simulink model "ModelSimulationOfTheRunningDeviationSystem"  (Simulink 8.9)
settings: Solver=VariableStepAuto  StartTime=0.0  StopTime=10.0  RelTol=1e-3
settings Model: Creator=xiang  LastModifiedBy=xiang
settings DataIOCC: LimitDataPoints=off  SaveFormat=Dataset  SignalLoggingSaveFormat=Dataset
settings OptimizationCC: LifeSpan=auto
settings DebuggingCC: UnderspecifiedInitializationDetection=Simplified  MergeDetectMultiDrivingBlocksExec=error  FcnCallInpInsideContextMsg=error  StateNameClashWarn=none  SFUnexpectedBacktrackingDiag=error  SFNoUnconditionalDefaultTransitionDiag=error  SFExecutionAtInitializationDiag=warning
settings HardwareCC: ProdBitPerPointer=64  ProdBitPerSizeT=64  ProdBitPerPtrDiffT=64  ProdLargestAtomicFloat=Float  ProdIntDivRoundTo=Zero  ProdEndianess=LittleEndian  ProdWordSize=64  ProdHWDeviceType=Intel->x86-64 (Windows64)
settings ModelReferenceCC: PropagateSignalLabelsOutOfModel=on
settings GRTTargetCC: TargetLangStandard=C99 (ISO)  GeneratePreprocessorConditionals=Use local settings  CombineOutputUpdateFcns=on  GRTInterface=off
settings ConfigComp: CovMetricSettings=dwe  CovHtmlReporting=off  CovSaveCumulativeToWorkspaceVar=off  CovSaveSingleToWorkspaceVar=off  CovExternalEMLEnable=on

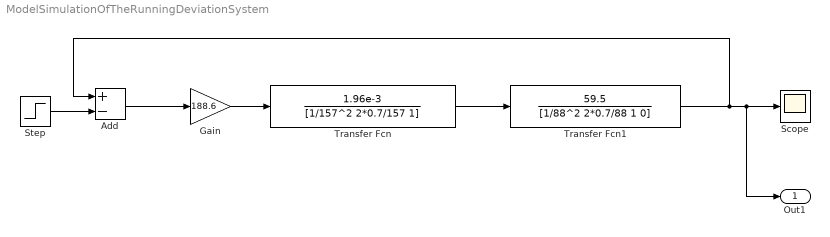
== system ModelSimulationOfTheRunningDeviationSystem ==
  Add : Sum  Inputs=+-
  Gain : Gain  Gain=188.6
  Scope : Scope
  Step : Step  SampleTime=0
  Transfer Fcn : TransferFcn  Numerator=[1.96e-3]  Denominator=[1/157^2 2*0.7/157 1]
  Transfer Fcn1 : TransferFcn  Numerator=[59.5]  Denominator=[1/88^2 2*0.7/88 1 0]
  Out1 : Outport
  wires:
  Gain/1 -> Transfer Fcn/1
  Add/1 -> Gain/1
  Transfer Fcn1/1 -> Add/1, Out1/1, Scope/1
  Step/1 -> Add/2
  Transfer Fcn/1 -> Transfer Fcn1/1
